simulink model "GPS_Constellation"  (R2018a)
settings: Solver=ode4  StartTime=0  StopTime=time_end  FixedStep=time_step  RelTol=1e-15  AbsTol=1e-15
values from neighbouring files (symbols this model uses):
  c = 299792458    [FFNAV_GPS_Params.mat]    (also in FFNAV_RunGPS.m; Test_GPS_Relativistic.m; Test_Klobuchar_Paper.m)
  GPS_COE = [4.6796815102 2.82369838363 0.203784643463 0.729652347089 1.65659671282 1.15813067845 3.02528391224 5.41010180216 3.56703411206 1.95260455396 0.205879038565 5.92829005708 ... (162 elements, 27x6)]    [FFNAV_GPS_Params.mat]    (also in FFNAV_RunGPS.m = [  268.126*deg2rad    SMA_GPS   ECC_GPS   INC_GPS   357.734*)
  mu = 398600441800000    [FFNAV_GPS_Params.mat]    (also in FFNAV_RunGPS.m; Test_GPS_Relativistic.m = 398600500000000)
undefined symbols (not defined in the file or in its folder): COE_chaser, COE_target
libraries: dspmtrx3 x27
(part 2 of 3)

== matlab function GPS_Constellation/GPS A1 /Orbital Mechanics/Orbital Mechanics ==
  data: v_ECI output; COE input; r_ECI output; mu parameter
 function [v_ECI,r_ECI] = Orb_Mech(COE, mu)
% ========================================================================
% Description: This funciton calculates the initial r and v vectors, 
% given the provided classiclal orbital elements defined in the
% initialization of the simulation.

%%========================================================================
%Extract COE values
theta       = COE(1);
a           = COE(2);
e           = COE(3);
i           = COE(4);
RAAN        = COE(5);
w           = COE(6);

%%========================================================================
r   = a*(1-e^2)/(1+e*cos(theta));                               %Defining the radius (Eq. 2.32)
p   = a*(1-e^2);                                                %Defining the semilatus rectum (Eq. 2.31)
r_P = [r*cos(theta) r*sin(theta) 0]';                           %(r in perifocal frame - Eq. 2.86) 
v_P = [-sqrt(mu/p)*sin(theta) sqrt(mu/p)*(e+cos(theta)) 0]';    %(v in perifocal frame - Eq. 2.87)

%Rotation Matrix from P to ECI Frame
C_IP = [    cos(RAAN)*cos(w)-sin(RAAN)*cos(i)*sin(w) -cos(RAAN)*sin(w)-sin(RAAN)*cos(i)*cos(w) sin(RAAN)*sin(i);
            sin(RAAN)*cos(w)+cos(RAAN)*cos(i)*sin(w) -sin(RAAN)*sin(w)+cos(RAAN)*cos(i)*cos(w) -cos(RAAN)*sin(i);
                        sin(i)*sin(w)                            sin(i)*cos(w)                       cos(i)  ];

%Definition of ECI Frame
x_ECI   = [1 0 0];
y_ECI   = [0 1 0];
z_ECI   = [0 0 1];
F_ECI   = [x_ECI; y_ECI; z_ECI]; %Reference Frame ECI

%r and v vectors in ECI Frame
r_ECI   = F_ECI*C_IP*r_P;
v_ECI   = F_ECI*C_IP*v_P;

%z_vec_ECI  = cross(r_ECI, v_ECI)/norm(cross(r_ECI, v_ECI));    %Check orientation of z vector
%X_ECI      = [r_ECI v_ECI]';                                   %State Vector in ECI components (Eq. 2.82)

r_mag = norm(r_ECI);
r_hat = r_ECI/r_mag;

end
% ========================================================================

== matlab function GPS_Constellation/GPS B1F/Orbital Mechanics/MATLAB Function1 ==
  data: r input; r_ddot output; mu input
function r_ddot = r_ddot(r, mu)
% ========================================================================
% Description: This function calculates -mu/r^3 *r to propagate the radius
% vector of the orbital motion

r_ddot = -(mu/(norm(r))^3)*r;

end
% ========================================================================

== matlab function GPS_Constellation/GPS B1F/Orbital Mechanics/Orbital Mechanics ==
  data: v_ECI output; COE input; r_ECI output; mu input
 function [v_ECI,r_ECI] = Orb_Mech(COE, mu)
% ========================================================================
% Description: This funciton calculates the initial r and v vectors, 
% given the provided classiclal orbital elements defined in the
% initialization of the simulation.

%%========================================================================
%Extract COE values
theta       = COE(1);
a           = COE(2);
e           = COE(3);
i           = COE(4);
RAAN        = COE(5);
w           = COE(6);

%%========================================================================
r   = a*(1-e^2)/(1+e*cos(theta));                               %Defining the radius (Eq. 2.32)
p   = a*(1-e^2);                                                %Defining the semilatus rectum (Eq. 2.31)
r_P = [r*cos(theta) r*sin(theta) 0]';                           %(r in perifocal frame - Eq. 2.86) 
v_P = [-sqrt(mu/p)*sin(theta) sqrt(mu/p)*(e+cos(theta)) 0]';    %(v in perifocal frame - Eq. 2.87)

%Rotation Matrix from P to ECI Frame
C_IP = [    cos(RAAN)*cos(w)-sin(RAAN)*cos(i)*sin(w) -cos(RAAN)*sin(w)-sin(RAAN)*cos(i)*cos(w) sin(RAAN)*sin(i);
            sin(RAAN)*cos(w)+cos(RAAN)*cos(i)*sin(w) -sin(RAAN)*sin(w)+cos(RAAN)*cos(i)*cos(w) -cos(RAAN)*sin(i);
                        sin(i)*sin(w)                            sin(i)*cos(w)                       cos(i)  ];

%Definition of ECI Frame
x_ECI   = [1 0 0];
y_ECI   = [0 1 0];
z_ECI   = [0 0 1];
F_ECI   = [x_ECI; y_ECI; z_ECI]; %Reference Frame ECI

%r and v vectors in ECI Frame
r_ECI   = F_ECI*C_IP*r_P;
v_ECI   = F_ECI*C_IP*v_P;

%z_vec_ECI  = cross(r_ECI, v_ECI)/norm(cross(r_ECI, v_ECI));    %Check orientation of z vector
%X_ECI      = [r_ECI v_ECI]';                                   %State Vector in ECI components (Eq. 2.82)

r_mag = norm(r_ECI);
r_hat = r_ECI/r_mag;

end
% ========================================================================

== matlab function GPS_Constellation/Orbital Mechanics for Target Spacecraft1/MATLAB Function1 ==
  data: r input; r_ddot output; mu parameter
function r_ddot = r_ddot(r, mu)
% ========================================================================
% Description: This function calculates -mu/r^3 *r to propagate the radius
% vector of the orbital motion

r_ddot = -(mu/(norm(r))^3)*r;

end
% ========================================================================

== matlab function GPS_Constellation/Orbital Mechanics for Target Spacecraft1/Target Orbital Mechanics ==
  data: v_ECI output; r_ECI output; mu parameter; COE_target parameter
 function [v_ECI,r_ECI] = Orb_Mech(mu, COE_target)
% ========================================================================
% Description: This funciton calculates the initial r and v vectors, 
% given the provided classiclal orbital elements defined in the
% initialization of the simulation.

%%========================================================================
%Extract COE values
theta       = COE_target(1);
a           = COE_target(2);
e           = COE_target(3);
i           = COE_target(4);
RAAN        = COE_target(5);
w           = COE_target(6);

%%========================================================================
r   = a*(1-e^2)/(1+e*cos(theta));                               %Defining the radius (Eq. 2.32)
p   = a*(1-e^2);                                                %Defining the semilatus rectum (Eq. 2.31)
r_P = [r*cos(theta) r*sin(theta) 0]';                           %(r in perifocal frame - Eq. 2.86) 
v_P = [-sqrt(mu/p)*sin(theta) sqrt(mu/p)*(e+cos(theta)) 0]';    %(v in perifocal frame - Eq. 2.87)

%Rotation Matrix from P to ECI Frame
C_IP = [    cos(RAAN)*cos(w)-sin(RAAN)*cos(i)*sin(w) -cos(RAAN)*sin(w)-sin(RAAN)*cos(i)*cos(w) sin(RAAN)*sin(i);
            sin(RAAN)*cos(w)+cos(RAAN)*cos(i)*sin(w) -sin(RAAN)*sin(w)+cos(RAAN)*cos(i)*cos(w) -cos(RAAN)*sin(i);
                        sin(i)*sin(w)                            sin(i)*cos(w)                       cos(i)  ];

%Definition of ECI Frame
x_ECI   = [1 0 0];
y_ECI   = [0 1 0];
z_ECI   = [0 0 1];
F_ECI   = [x_ECI; y_ECI; z_ECI]; %Reference Frame ECI

%r and v vectors in ECI Frame
r_ECI   = F_ECI*C_IP*r_P;
v_ECI   = F_ECI*C_IP*v_P;

%z_vec_ECI  = cross(r_ECI, v_ECI)/norm(cross(r_ECI, v_ECI));    %Check orientation of z vector
%X_ECI      = [r_ECI v_ECI]';                                   %State Vector in ECI components (Eq. 2.82)

r_mag = norm(r_ECI);
r_hat = r_ECI/r_mag;

end
% ========================================================================

== matlab function GPS_Constellation/GPS A3/Orbital Mechanics/MATLAB Function1 ==
  data: r input; r_ddot output; mu input
function r_ddot = r_ddot(r, mu)
% ========================================================================
% Description: This function calculates -mu/r^3 *r to propagate the radius
% vector of the orbital motion

r_ddot = -(mu/(norm(r))^3)*r;

end
% ========================================================================

== matlab function GPS_Constellation/GPS A3/Orbital Mechanics/Orbital Mechanics ==
  data: v_ECI output; COE input; r_ECI output; mu input
 function [v_ECI,r_ECI] = Orb_Mech(COE, mu)
% ========================================================================
% Description: This funciton calculates the initial r and v vectors, 
% given the provided classiclal orbital elements defined in the
% initialization of the simulation.

%%========================================================================
%Extract COE values
theta       = COE(1);
a           = COE(2);
e           = COE(3);
i           = COE(4);
RAAN        = COE(5);
w           = COE(6);

%%========================================================================
r   = a*(1-e^2)/(1+e*cos(theta));                               %Defining the radius (Eq. 2.32)
p   = a*(1-e^2);                                                %Defining the semilatus rectum (Eq. 2.31)
r_P = [r*cos(theta) r*sin(theta) 0]';                           %(r in perifocal frame - Eq. 2.86) 
v_P = [-sqrt(mu/p)*sin(theta) sqrt(mu/p)*(e+cos(theta)) 0]';    %(v in perifocal frame - Eq. 2.87)

%Rotation Matrix from P to ECI Frame
C_IP = [    cos(RAAN)*cos(w)-sin(RAAN)*cos(i)*sin(w) -cos(RAAN)*sin(w)-sin(RAAN)*cos(i)*cos(w) sin(RAAN)*sin(i);
            sin(RAAN)*cos(w)+cos(RAAN)*cos(i)*sin(w) -sin(RAAN)*sin(w)+cos(RAAN)*cos(i)*cos(w) -cos(RAAN)*sin(i);
                        sin(i)*sin(w)                            sin(i)*cos(w)                       cos(i)  ];

%Definition of ECI Frame
x_ECI   = [1 0 0];
y_ECI   = [0 1 0];
z_ECI   = [0 0 1];
F_ECI   = [x_ECI; y_ECI; z_ECI]; %Reference Frame ECI

%r and v vectors in ECI Frame
r_ECI   = F_ECI*C_IP*r_P;
v_ECI   = F_ECI*C_IP*v_P;

%z_vec_ECI  = cross(r_ECI, v_ECI)/norm(cross(r_ECI, v_ECI));    %Check orientation of z vector
%X_ECI      = [r_ECI v_ECI]';                                   %State Vector in ECI components (Eq. 2.82)

r_mag = norm(r_ECI);
r_hat = r_ECI/r_mag;

end
% ========================================================================

== matlab function GPS_Constellation/GPS A4/Orbital Mechanics/MATLAB Function1 ==
  data: r input; r_ddot output; mu input
function r_ddot = r_ddot(r, mu)
% ========================================================================
% Description: This function calculates -mu/r^3 *r to propagate the radius
% vector of the orbital motion

r_ddot = -(mu/(norm(r))^3)*r;

end
% ========================================================================

== matlab function GPS_Constellation/GPS A4/Orbital Mechanics/Orbital Mechanics ==
  data: v_ECI output; COE input; r_ECI output; mu input
 function [v_ECI,r_ECI] = Orb_Mech(COE, mu)
% ========================================================================
% Description: This funciton calculates the initial r and v vectors, 
% given the provided classiclal orbital elements defined in the
% initialization of the simulation.

%%========================================================================
%Extract COE values
theta       = COE(1);
a           = COE(2);
e           = COE(3);
i           = COE(4);
RAAN        = COE(5);
w           = COE(6);

%%========================================================================
r   = a*(1-e^2)/(1+e*cos(theta));                               %Defining the radius (Eq. 2.32)
p   = a*(1-e^2);                                                %Defining the semilatus rectum (Eq. 2.31)
r_P = [r*cos(theta) r*sin(theta) 0]';                           %(r in perifocal frame - Eq. 2.86) 
v_P = [-sqrt(mu/p)*sin(theta) sqrt(mu/p)*(e+cos(theta)) 0]';    %(v in perifocal frame - Eq. 2.87)

%Rotation Matrix from P to ECI Frame
C_IP = [    cos(RAAN)*cos(w)-sin(RAAN)*cos(i)*sin(w) -cos(RAAN)*sin(w)-sin(RAAN)*cos(i)*cos(w) sin(RAAN)*sin(i);
            sin(RAAN)*cos(w)+cos(RAAN)*cos(i)*sin(w) -sin(RAAN)*sin(w)+cos(RAAN)*cos(i)*cos(w) -cos(RAAN)*sin(i);
                        sin(i)*sin(w)                            sin(i)*cos(w)                       cos(i)  ];

%Definition of ECI Frame
x_ECI   = [1 0 0];
y_ECI   = [0 1 0];
z_ECI   = [0 0 1];
F_ECI   = [x_ECI; y_ECI; z_ECI]; %Reference Frame ECI

%r and v vectors in ECI Frame
r_ECI   = F_ECI*C_IP*r_P;
v_ECI   = F_ECI*C_IP*v_P;

%z_vec_ECI  = cross(r_ECI, v_ECI)/norm(cross(r_ECI, v_ECI));    %Check orientation of z vector
%X_ECI      = [r_ECI v_ECI]';                                   %State Vector in ECI components (Eq. 2.82)

r_mag = norm(r_ECI);
r_hat = r_ECI/r_mag;

end
% ========================================================================

== matlab function GPS_Constellation/GPS B1A/Orbital Mechanics/MATLAB Function1 ==
  data: r input; r_ddot output; mu input
function r_ddot = r_ddot(r, mu)
% ========================================================================
% Description: This function calculates -mu/r^3 *r to propagate the radius
% vector of the orbital motion

r_ddot = -(mu/(norm(r))^3)*r;

end
% ========================================================================

== matlab function GPS_Constellation/GPS B1A/Orbital Mechanics/Orbital Mechanics ==
  data: v_ECI output; COE input; r_ECI output; mu input
 function [v_ECI,r_ECI] = Orb_Mech(COE, mu)
% ========================================================================
% Description: This funciton calculates the initial r and v vectors, 
% given the provided classiclal orbital elements defined in the
% initialization of the simulation.

%%========================================================================
%Extract COE values
theta       = COE(1);
a           = COE(2);
e           = COE(3);
i           = COE(4);
RAAN        = COE(5);
w           = COE(6);

%%========================================================================
r   = a*(1-e^2)/(1+e*cos(theta));                               %Defining the radius (Eq. 2.32)
p   = a*(1-e^2);                                                %Defining the semilatus rectum (Eq. 2.31)
r_P = [r*cos(theta) r*sin(theta) 0]';                           %(r in perifocal frame - Eq. 2.86) 
v_P = [-sqrt(mu/p)*sin(theta) sqrt(mu/p)*(e+cos(theta)) 0]';    %(v in perifocal frame - Eq. 2.87)

%Rotation Matrix from P to ECI Frame
C_IP = [    cos(RAAN)*cos(w)-sin(RAAN)*cos(i)*sin(w) -cos(RAAN)*sin(w)-sin(RAAN)*cos(i)*cos(w) sin(RAAN)*sin(i);
            sin(RAAN)*cos(w)+cos(RAAN)*cos(i)*sin(w) -sin(RAAN)*sin(w)+cos(RAAN)*cos(i)*cos(w) -cos(RAAN)*sin(i);
                        sin(i)*sin(w)                            sin(i)*cos(w)                       cos(i)  ];

%Definition of ECI Frame
x_ECI   = [1 0 0];
y_ECI   = [0 1 0];
z_ECI   = [0 0 1];
F_ECI   = [x_ECI; y_ECI; z_ECI]; %Reference Frame ECI

%r and v vectors in ECI Frame
r_ECI   = F_ECI*C_IP*r_P;
v_ECI   = F_ECI*C_IP*v_P;

%z_vec_ECI  = cross(r_ECI, v_ECI)/norm(cross(r_ECI, v_ECI));    %Check orientation of z vector
%X_ECI      = [r_ECI v_ECI]';                                   %State Vector in ECI components (Eq. 2.82)

r_mag = norm(r_ECI);
r_hat = r_ECI/r_mag;

end
% ========================================================================

== matlab function GPS_Constellation/GPS B2/Orbital Mechanics/MATLAB Function1 ==
  data: r input; r_ddot output; mu input
function r_ddot = r_ddot(r, mu)
% ========================================================================
% Description: This function calculates -mu/r^3 *r to propagate the radius
% vector of the orbital motion

r_ddot = -(mu/(norm(r))^3)*r;

end
% ========================================================================

== matlab function GPS_Constellation/GPS B2/Orbital Mechanics/Orbital Mechanics ==
  data: v_ECI output; COE input; r_ECI output; mu input
 function [v_ECI,r_ECI] = Orb_Mech(COE, mu)
% ========================================================================
% Description: This funciton calculates the initial r and v vectors, 
% given the provided classiclal orbital elements defined in the
% initialization of the simulation.

%%========================================================================
%Extract COE values
theta       = COE(1);
a           = COE(2);
e           = COE(3);
i           = COE(4);
RAAN        = COE(5);
w           = COE(6);

%%========================================================================
r   = a*(1-e^2)/(1+e*cos(theta));                               %Defining the radius (Eq. 2.32)
p   = a*(1-e^2);                                                %Defining the semilatus rectum (Eq. 2.31)
r_P = [r*cos(theta) r*sin(theta) 0]';                           %(r in perifocal frame - Eq. 2.86) 
v_P = [-sqrt(mu/p)*sin(theta) sqrt(mu/p)*(e+cos(theta)) 0]';    %(v in perifocal frame - Eq. 2.87)

%Rotation Matrix from P to ECI Frame
C_IP = [    cos(RAAN)*cos(w)-sin(RAAN)*cos(i)*sin(w) -cos(RAAN)*sin(w)-sin(RAAN)*cos(i)*cos(w) sin(RAAN)*sin(i);
            sin(RAAN)*cos(w)+cos(RAAN)*cos(i)*sin(w) -sin(RAAN)*sin(w)+cos(RAAN)*cos(i)*cos(w) -cos(RAAN)*sin(i);
                        sin(i)*sin(w)                            sin(i)*cos(w)                       cos(i)  ];

%Definition of ECI Frame
x_ECI   = [1 0 0];
y_ECI   = [0 1 0];
z_ECI   = [0 0 1];
F_ECI   = [x_ECI; y_ECI; z_ECI]; %Reference Frame ECI

%r and v vectors in ECI Frame
r_ECI   = F_ECI*C_IP*r_P;
v_ECI   = F_ECI*C_IP*v_P;

%z_vec_ECI  = cross(r_ECI, v_ECI)/norm(cross(r_ECI, v_ECI));    %Check orientation of z vector
%X_ECI      = [r_ECI v_ECI]';                                   %State Vector in ECI components (Eq. 2.82)

r_mag = norm(r_ECI);
r_hat = r_ECI/r_mag;

end
% ========================================================================

== matlab function GPS_Constellation/GPS B3/Orbital Mechanics/MATLAB Function1 ==
  data: r input; r_ddot output; mu input
function r_ddot = r_ddot(r, mu)
% ========================================================================
% Description: This function calculates -mu/r^3 *r to propagate the radius
% vector of the orbital motion

r_ddot = -(mu/(norm(r))^3)*r;

end
% ========================================================================

== matlab function GPS_Constellation/GPS B3/Orbital Mechanics/Orbital Mechanics ==
  data: v_ECI output; COE input; r_ECI output; mu input
 function [v_ECI,r_ECI] = Orb_Mech(COE, mu)
% ========================================================================
% Description: This funciton calculates the initial r and v vectors, 
% given the provided classiclal orbital elements defined in the
% initialization of the simulation.

%%========================================================================
%Extract COE values
theta       = COE(1);
a           = COE(2);
e           = COE(3);
i           = COE(4);
RAAN        = COE(5);
w           = COE(6);

%%========================================================================
r   = a*(1-e^2)/(1+e*cos(theta));                               %Defining the radius (Eq. 2.32)
p   = a*(1-e^2);                                                %Defining the semilatus rectum (Eq. 2.31)
r_P = [r*cos(theta) r*sin(theta) 0]';                           %(r in perifocal frame - Eq. 2.86) 
v_P = [-sqrt(mu/p)*sin(theta) sqrt(mu/p)*(e+cos(theta)) 0]';    %(v in perifocal frame - Eq. 2.87)

%Rotation Matrix from P to ECI Frame
C_IP = [    cos(RAAN)*cos(w)-sin(RAAN)*cos(i)*sin(w) -cos(RAAN)*sin(w)-sin(RAAN)*cos(i)*cos(w) sin(RAAN)*sin(i);
            sin(RAAN)*cos(w)+cos(RAAN)*cos(i)*sin(w) -sin(RAAN)*sin(w)+cos(RAAN)*cos(i)*cos(w) -cos(RAAN)*sin(i);
                        sin(i)*sin(w)                            sin(i)*cos(w)                       cos(i)  ];

%Definition of ECI Frame
x_ECI   = [1 0 0];
y_ECI   = [0 1 0];
z_ECI   = [0 0 1];
F_ECI   = [x_ECI; y_ECI; z_ECI]; %Reference Frame ECI

%r and v vectors in ECI Frame
r_ECI   = F_ECI*C_IP*r_P;
v_ECI   = F_ECI*C_IP*v_P;

%z_vec_ECI  = cross(r_ECI, v_ECI)/norm(cross(r_ECI, v_ECI));    %Check orientation of z vector
%X_ECI      = [r_ECI v_ECI]';                                   %State Vector in ECI components (Eq. 2.82)

r_mag = norm(r_ECI);
r_hat = r_ECI/r_mag;

end
% ========================================================================

== matlab function GPS_Constellation/GPS B4/Orbital Mechanics/MATLAB Function1 ==
  data: r input; r_ddot output; mu input
function r_ddot = r_ddot(r, mu)
% ========================================================================
% Description: This function calculates -mu/r^3 *r to propagate the radius
% vector of the orbital motion

r_ddot = -(mu/(norm(r))^3)*r;

end
% ========================================================================

== matlab function GPS_Constellation/GPS B4/Orbital Mechanics/Orbital Mechanics ==
  data: v_ECI output; COE input; r_ECI output; mu input
 function [v_ECI,r_ECI] = Orb_Mech(COE, mu)
% ========================================================================
% Description: This funciton calculates the initial r and v vectors, 
% given the provided classiclal orbital elements defined in the
% initialization of the simulation.

%%========================================================================
%Extract COE values
theta       = COE(1);
a           = COE(2);
e           = COE(3);
i           = COE(4);
RAAN        = COE(5);
w           = COE(6);

%%========================================================================
r   = a*(1-e^2)/(1+e*cos(theta));                               %Defining the radius (Eq. 2.32)
p   = a*(1-e^2);                                                %Defining the semilatus rectum (Eq. 2.31)
r_P = [r*cos(theta) r*sin(theta) 0]';                           %(r in perifocal frame - Eq. 2.86) 
v_P = [-sqrt(mu/p)*sin(theta) sqrt(mu/p)*(e+cos(theta)) 0]';    %(v in perifocal frame - Eq. 2.87)

%Rotation Matrix from P to ECI Frame
C_IP = [    cos(RAAN)*cos(w)-sin(RAAN)*cos(i)*sin(w) -cos(RAAN)*sin(w)-sin(RAAN)*cos(i)*cos(w) sin(RAAN)*sin(i);
            sin(RAAN)*cos(w)+cos(RAAN)*cos(i)*sin(w) -sin(RAAN)*sin(w)+cos(RAAN)*cos(i)*cos(w) -cos(RAAN)*sin(i);
                        sin(i)*sin(w)                            sin(i)*cos(w)                       cos(i)  ];

%Definition of ECI Frame
x_ECI   = [1 0 0];
y_ECI   = [0 1 0];
z_ECI   = [0 0 1];
F_ECI   = [x_ECI; y_ECI; z_ECI]; %Reference Frame ECI

%r and v vectors in ECI Frame
r_ECI   = F_ECI*C_IP*r_P;
v_ECI   = F_ECI*C_IP*v_P;

%z_vec_ECI  = cross(r_ECI, v_ECI)/norm(cross(r_ECI, v_ECI));    %Check orientation of z vector
%X_ECI      = [r_ECI v_ECI]';                                   %State Vector in ECI components (Eq. 2.82)

r_mag = norm(r_ECI);
r_hat = r_ECI/r_mag;

end
% ========================================================================

== matlab function GPS_Constellation/GPS C3/Orbital Mechanics/MATLAB Function1 ==
  data: r input; r_ddot output; mu input
function r_ddot = r_ddot(r, mu)
% ========================================================================
% Description: This function calculates -mu/r^3 *r to propagate the radius
% vector of the orbital motion

r_ddot = -(mu/(norm(r))^3)*r;

end
% ========================================================================

== matlab function GPS_Constellation/GPS C3/Orbital Mechanics/Orbital Mechanics ==
  data: v_ECI output; COE input; r_ECI output; mu input
 function [v_ECI,r_ECI] = Orb_Mech(COE, mu)
% ========================================================================
% Description: This funciton calculates the initial r and v vectors, 
% given the provided classiclal orbital elements defined in the
% initialization of the simulation.

%%========================================================================
%Extract COE values
theta       = COE(1);
a           = COE(2);
e           = COE(3);
i           = COE(4);
RAAN        = COE(5);
w           = COE(6);

%%========================================================================
r   = a*(1-e^2)/(1+e*cos(theta));                               %Defining the radius (Eq. 2.32)
p   = a*(1-e^2);                                                %Defining the semilatus rectum (Eq. 2.31)
r_P = [r*cos(theta) r*sin(theta) 0]';                           %(r in perifocal frame - Eq. 2.86) 
v_P = [-sqrt(mu/p)*sin(theta) sqrt(mu/p)*(e+cos(theta)) 0]';    %(v in perifocal frame - Eq. 2.87)

%Rotation Matrix from P to ECI Frame
C_IP = [    cos(RAAN)*cos(w)-sin(RAAN)*cos(i)*sin(w) -cos(RAAN)*sin(w)-sin(RAAN)*cos(i)*cos(w) sin(RAAN)*sin(i);
            sin(RAAN)*cos(w)+cos(RAAN)*cos(i)*sin(w) -sin(RAAN)*sin(w)+cos(RAAN)*cos(i)*cos(w) -cos(RAAN)*sin(i);
                        sin(i)*sin(w)                            sin(i)*cos(w)                       cos(i)  ];

%Definition of ECI Frame
x_ECI   = [1 0 0];
y_ECI   = [0 1 0];
z_ECI   = [0 0 1];
F_ECI   = [x_ECI; y_ECI; z_ECI]; %Reference Frame ECI

%r and v vectors in ECI Frame
r_ECI   = F_ECI*C_IP*r_P;
v_ECI   = F_ECI*C_IP*v_P;

%z_vec_ECI  = cross(r_ECI, v_ECI)/norm(cross(r_ECI, v_ECI));    %Check orientation of z vector
%X_ECI      = [r_ECI v_ECI]';                                   %State Vector in ECI components (Eq. 2.82)

r_mag = norm(r_ECI);
r_hat = r_ECI/r_mag;

end
% ========================================================================

== matlab function GPS_Constellation/GPS C2/Orbital Mechanics/MATLAB Function1 ==
  data: r input; r_ddot output; mu input
function r_ddot = r_ddot(r, mu)
% ========================================================================
% Description: This function calculates -mu/r^3 *r to propagate the radius
% vector of the orbital motion

r_ddot = -(mu/(norm(r))^3)*r;

end
% ========================================================================

== matlab function GPS_Constellation/GPS C2/Orbital Mechanics/Orbital Mechanics ==
  data: v_ECI output; COE input; r_ECI output; mu input
 function [v_ECI,r_ECI] = Orb_Mech(COE, mu)
% ========================================================================
% Description: This funciton calculates the initial r and v vectors, 
% given the provided classiclal orbital elements defined in the
% initialization of the simulation.

%%========================================================================
%Extract COE values
theta       = COE(1);
a           = COE(2);
e           = COE(3);
i           = COE(4);
RAAN        = COE(5);
w           = COE(6);

%%========================================================================
r   = a*(1-e^2)/(1+e*cos(theta));                               %Defining the radius (Eq. 2.32)
p   = a*(1-e^2);                                                %Defining the semilatus rectum (Eq. 2.31)
r_P = [r*cos(theta) r*sin(theta) 0]';                           %(r in perifocal frame - Eq. 2.86) 
v_P = [-sqrt(mu/p)*sin(theta) sqrt(mu/p)*(e+cos(theta)) 0]';    %(v in perifocal frame - Eq. 2.87)

%Rotation Matrix from P to ECI Frame
C_IP = [    cos(RAAN)*cos(w)-sin(RAAN)*cos(i)*sin(w) -cos(RAAN)*sin(w)-sin(RAAN)*cos(i)*cos(w) sin(RAAN)*sin(i);
            sin(RAAN)*cos(w)+cos(RAAN)*cos(i)*sin(w) -sin(RAAN)*sin(w)+cos(RAAN)*cos(i)*cos(w) -cos(RAAN)*sin(i);
                        sin(i)*sin(w)                            sin(i)*cos(w)                       cos(i)  ];

%Definition of ECI Frame
x_ECI   = [1 0 0];
y_ECI   = [0 1 0];
z_ECI   = [0 0 1];
F_ECI   = [x_ECI; y_ECI; z_ECI]; %Reference Frame ECI

%r and v vectors in ECI Frame
r_ECI   = F_ECI*C_IP*r_P;
v_ECI   = F_ECI*C_IP*v_P;

%z_vec_ECI  = cross(r_ECI, v_ECI)/norm(cross(r_ECI, v_ECI));    %Check orientation of z vector
%X_ECI      = [r_ECI v_ECI]';                                   %State Vector in ECI components (Eq. 2.82)

r_mag = norm(r_ECI);
r_hat = r_ECI/r_mag;

end
% ========================================================================

== matlab function GPS_Constellation/GPS C1/Orbital Mechanics/MATLAB Function1 ==
  data: r input; r_ddot output; mu input
function r_ddot = r_ddot(r, mu)
% ========================================================================
% Description: This function calculates -mu/r^3 *r to propagate the radius
% vector of the orbital motion

r_ddot = -(mu/(norm(r))^3)*r;

end
% ========================================================================

== matlab function GPS_Constellation/GPS C1/Orbital Mechanics/Orbital Mechanics ==
  data: v_ECI output; COE input; r_ECI output; mu input
 function [v_ECI,r_ECI] = Orb_Mech(COE, mu)
% ========================================================================
% Description: This funciton calculates the initial r and v vectors, 
% given the provided classiclal orbital elements defined in the
% initialization of the simulation.

%%========================================================================
%Extract COE values
theta       = COE(1);
a           = COE(2);
e           = COE(3);
i           = COE(4);
RAAN        = COE(5);
w           = COE(6);

%%========================================================================
r   = a*(1-e^2)/(1+e*cos(theta));                               %Defining the radius (Eq. 2.32)
p   = a*(1-e^2);                                                %Defining the semilatus rectum (Eq. 2.31)
r_P = [r*cos(theta) r*sin(theta) 0]';                           %(r in perifocal frame - Eq. 2.86) 
v_P = [-sqrt(mu/p)*sin(theta) sqrt(mu/p)*(e+cos(theta)) 0]';    %(v in perifocal frame - Eq. 2.87)

%Rotation Matrix from P to ECI Frame
C_IP = [    cos(RAAN)*cos(w)-sin(RAAN)*cos(i)*sin(w) -cos(RAAN)*sin(w)-sin(RAAN)*cos(i)*cos(w) sin(RAAN)*sin(i);
            sin(RAAN)*cos(w)+cos(RAAN)*cos(i)*sin(w) -sin(RAAN)*sin(w)+cos(RAAN)*cos(i)*cos(w) -cos(RAAN)*sin(i);
                        sin(i)*sin(w)                            sin(i)*cos(w)                       cos(i)  ];

%Definition of ECI Frame
x_ECI   = [1 0 0];
y_ECI   = [0 1 0];
z_ECI   = [0 0 1];
F_ECI   = [x_ECI; y_ECI; z_ECI]; %Reference Frame ECI

%r and v vectors in ECI Frame
r_ECI   = F_ECI*C_IP*r_P;
v_ECI   = F_ECI*C_IP*v_P;

%z_vec_ECI  = cross(r_ECI, v_ECI)/norm(cross(r_ECI, v_ECI));    %Check orientation of z vector
%X_ECI      = [r_ECI v_ECI]';                                   %State Vector in ECI components (Eq. 2.82)

r_mag = norm(r_ECI);
r_hat = r_ECI/r_mag;

end
% ========================================================================

== matlab function GPS_Constellation/GPS C4/Orbital Mechanics/MATLAB Function1 ==
  data: r input; r_ddot output; mu input
function r_ddot = r_ddot(r, mu)
% ========================================================================
% Description: This function calculates -mu/r^3 *r to propagate the radius
% vector of the orbital motion

r_ddot = -(mu/(norm(r))^3)*r;

end
% ========================================================================

== matlab function GPS_Constellation/GPS C4/Orbital Mechanics/Orbital Mechanics ==
  data: v_ECI output; COE input; r_ECI output; mu input
 function [v_ECI,r_ECI] = Orb_Mech(COE, mu)
% ========================================================================
% Description: This funciton calculates the initial r and v vectors, 
% given the provided classiclal orbital elements defined in the
% initialization of the simulation.

%%========================================================================
%Extract COE values
theta       = COE(1);
a           = COE(2);
e           = COE(3);
i           = COE(4);
RAAN        = COE(5);
w           = COE(6);

%%========================================================================
r   = a*(1-e^2)/(1+e*cos(theta));                               %Defining the radius (Eq. 2.32)
p   = a*(1-e^2);                                                %Defining the semilatus rectum (Eq. 2.31)
r_P = [r*cos(theta) r*sin(theta) 0]';                           %(r in perifocal frame - Eq. 2.86) 
v_P = [-sqrt(mu/p)*sin(theta) sqrt(mu/p)*(e+cos(theta)) 0]';    %(v in perifocal frame - Eq. 2.87)

%Rotation Matrix from P to ECI Frame
C_IP = [    cos(RAAN)*cos(w)-sin(RAAN)*cos(i)*sin(w) -cos(RAAN)*sin(w)-sin(RAAN)*cos(i)*cos(w) sin(RAAN)*sin(i);
            sin(RAAN)*cos(w)+cos(RAAN)*cos(i)*sin(w) -sin(RAAN)*sin(w)+cos(RAAN)*cos(i)*cos(w) -cos(RAAN)*sin(i);
                        sin(i)*sin(w)                            sin(i)*cos(w)                       cos(i)  ];

%Definition of ECI Frame
x_ECI   = [1 0 0];
y_ECI   = [0 1 0];
z_ECI   = [0 0 1];
F_ECI   = [x_ECI; y_ECI; z_ECI]; %Reference Frame ECI

%r and v vectors in ECI Frame
r_ECI   = F_ECI*C_IP*r_P;
v_ECI   = F_ECI*C_IP*v_P;

%z_vec_ECI  = cross(r_ECI, v_ECI)/norm(cross(r_ECI, v_ECI));    %Check orientation of z vector
%X_ECI      = [r_ECI v_ECI]';                                   %State Vector in ECI components (Eq. 2.82)

r_mag = norm(r_ECI);
r_hat = r_ECI/r_mag;

end
% ========================================================================

== matlab function GPS_Constellation/GPS D2A/Orbital Mechanics/MATLAB Function1 ==
  data: r input; r_ddot output; mu input
function r_ddot = r_ddot(r, mu)
% ========================================================================
% Description: This function calculates -mu/r^3 *r to propagate the radius
% vector of the orbital motion

r_ddot = -(mu/(norm(r))^3)*r;

end
% ========================================================================

== matlab function GPS_Constellation/GPS D2A/Orbital Mechanics/Orbital Mechanics ==
  data: v_ECI output; COE input; r_ECI output; mu input
 function [v_ECI,r_ECI] = Orb_Mech(COE, mu)
% ========================================================================
% Description: This funciton calculates the initial r and v vectors, 
% given the provided classiclal orbital elements defined in the
% initialization of the simulation.

%%========================================================================
%Extract COE values
theta       = COE(1);
a           = COE(2);
e           = COE(3);
i           = COE(4);
RAAN        = COE(5);
w           = COE(6);

%%========================================================================
r   = a*(1-e^2)/(1+e*cos(theta));                               %Defining the radius (Eq. 2.32)
p   = a*(1-e^2);                                                %Defining the semilatus rectum (Eq. 2.31)
r_P = [r*cos(theta) r*sin(theta) 0]';                           %(r in perifocal frame - Eq. 2.86) 
v_P = [-sqrt(mu/p)*sin(theta) sqrt(mu/p)*(e+cos(theta)) 0]';    %(v in perifocal frame - Eq. 2.87)

%Rotation Matrix from P to ECI Frame
C_IP = [    cos(RAAN)*cos(w)-sin(RAAN)*cos(i)*sin(w) -cos(RAAN)*sin(w)-sin(RAAN)*cos(i)*cos(w) sin(RAAN)*sin(i);
            sin(RAAN)*cos(w)+cos(RAAN)*cos(i)*sin(w) -sin(RAAN)*sin(w)+cos(RAAN)*cos(i)*cos(w) -cos(RAAN)*sin(i);
                        sin(i)*sin(w)                            sin(i)*cos(w)                       cos(i)  ];

%Definition of ECI Frame
x_ECI   = [1 0 0];
y_ECI   = [0 1 0];
z_ECI   = [0 0 1];
F_ECI   = [x_ECI; y_ECI; z_ECI]; %Reference Frame ECI

%r and v vectors in ECI Frame
r_ECI   = F_ECI*C_IP*r_P;
v_ECI   = F_ECI*C_IP*v_P;

%z_vec_ECI  = cross(r_ECI, v_ECI)/norm(cross(r_ECI, v_ECI));    %Check orientation of z vector
%X_ECI      = [r_ECI v_ECI]';                                   %State Vector in ECI components (Eq. 2.82)

r_mag = norm(r_ECI);
r_hat = r_ECI/r_mag;

end
% ========================================================================

== matlab function GPS_Constellation/GPS D2F/Orbital Mechanics/MATLAB Function1 ==
  data: r input; r_ddot output; mu input
function r_ddot = r_ddot(r, mu)
% ========================================================================
% Description: This function calculates -mu/r^3 *r to propagate the radius
% vector of the orbital motion

r_ddot = -(mu/(norm(r))^3)*r;

end
% ========================================================================

== matlab function GPS_Constellation/GPS D2F/Orbital Mechanics/Orbital Mechanics ==
  data: v_ECI output; COE input; r_ECI output; mu input
 function [v_ECI,r_ECI] = Orb_Mech(COE, mu)
% ========================================================================
% Description: This funciton calculates the initial r and v vectors, 
% given the provided classiclal orbital elements defined in the
% initialization of the simulation.

%%========================================================================
%Extract COE values
theta       = COE(1);
a           = COE(2);
e           = COE(3);
i           = COE(4);
RAAN        = COE(5);
w           = COE(6);

%%========================================================================
r   = a*(1-e^2)/(1+e*cos(theta));                               %Defining the radius (Eq. 2.32)
p   = a*(1-e^2);                                                %Defining the semilatus rectum (Eq. 2.31)
r_P = [r*cos(theta) r*sin(theta) 0]';                           %(r in perifocal frame - Eq. 2.86) 
v_P = [-sqrt(mu/p)*sin(theta) sqrt(mu/p)*(e+cos(theta)) 0]';    %(v in perifocal frame - Eq. 2.87)

%Rotation Matrix from P to ECI Frame
C_IP = [    cos(RAAN)*cos(w)-sin(RAAN)*cos(i)*sin(w) -cos(RAAN)*sin(w)-sin(RAAN)*cos(i)*cos(w) sin(RAAN)*sin(i);
            sin(RAAN)*cos(w)+cos(RAAN)*cos(i)*sin(w) -sin(RAAN)*sin(w)+cos(RAAN)*cos(i)*cos(w) -cos(RAAN)*sin(i);
                        sin(i)*sin(w)                            sin(i)*cos(w)                       cos(i)  ];

%Definition of ECI Frame
x_ECI   = [1 0 0];
y_ECI   = [0 1 0];
z_ECI   = [0 0 1];
F_ECI   = [x_ECI; y_ECI; z_ECI]; %Reference Frame ECI

%r and v vectors in ECI Frame
r_ECI   = F_ECI*C_IP*r_P;
v_ECI   = F_ECI*C_IP*v_P;

%z_vec_ECI  = cross(r_ECI, v_ECI)/norm(cross(r_ECI, v_ECI));    %Check orientation of z vector
%X_ECI      = [r_ECI v_ECI]';                                   %State Vector in ECI components (Eq. 2.82)

r_mag = norm(r_ECI);
r_hat = r_ECI/r_mag;

end
% ========================================================================

== matlab function GPS_Constellation/GPS D1/Orbital Mechanics/MATLAB Function1 ==
  data: r input; r_ddot output; mu input
function r_ddot = r_ddot(r, mu)
% ========================================================================
% Description: This function calculates -mu/r^3 *r to propagate the radius
% vector of the orbital motion

r_ddot = -(mu/(norm(r))^3)*r;

end
% ========================================================================

== matlab function GPS_Constellation/GPS D1/Orbital Mechanics/Orbital Mechanics ==
  data: v_ECI output; COE input; r_ECI output; mu input
 function [v_ECI,r_ECI] = Orb_Mech(COE, mu)
% ========================================================================
% Description: This funciton calculates the initial r and v vectors, 
% given the provided classiclal orbital elements defined in the
% initialization of the simulation.

%%========================================================================
%Extract COE values
theta       = COE(1);
a           = COE(2);
e           = COE(3);
i           = COE(4);
RAAN        = COE(5);
w           = COE(6);

%%========================================================================
r   = a*(1-e^2)/(1+e*cos(theta));                               %Defining the radius (Eq. 2.32)
p   = a*(1-e^2);                                                %Defining the semilatus rectum (Eq. 2.31)
r_P = [r*cos(theta) r*sin(theta) 0]';                           %(r in perifocal frame - Eq. 2.86) 
v_P = [-sqrt(mu/p)*sin(theta) sqrt(mu/p)*(e+cos(theta)) 0]';    %(v in perifocal frame - Eq. 2.87)

%Rotation Matrix from P to ECI Frame
C_IP = [    cos(RAAN)*cos(w)-sin(RAAN)*cos(i)*sin(w) -cos(RAAN)*sin(w)-sin(RAAN)*cos(i)*cos(w) sin(RAAN)*sin(i);
            sin(RAAN)*cos(w)+cos(RAAN)*cos(i)*sin(w) -sin(RAAN)*sin(w)+cos(RAAN)*cos(i)*cos(w) -cos(RAAN)*sin(i);
                        sin(i)*sin(w)                            sin(i)*cos(w)                       cos(i)  ];

%Definition of ECI Frame
x_ECI   = [1 0 0];
y_ECI   = [0 1 0];
z_ECI   = [0 0 1];
F_ECI   = [x_ECI; y_ECI; z_ECI]; %Reference Frame ECI

%r and v vectors in ECI Frame
r_ECI   = F_ECI*C_IP*r_P;
v_ECI   = F_ECI*C_IP*v_P;

%z_vec_ECI  = cross(r_ECI, v_ECI)/norm(cross(r_ECI, v_ECI));    %Check orientation of z vector
%X_ECI      = [r_ECI v_ECI]';                                   %State Vector in ECI components (Eq. 2.82)

r_mag = norm(r_ECI);
r_hat = r_ECI/r_mag;

end
% ========================================================================

== matlab function GPS_Constellation/GPS D3/Orbital Mechanics/MATLAB Function1 ==
  data: r input; r_ddot output; mu input
function r_ddot = r_ddot(r, mu)
% ========================================================================
% Description: This function calculates -mu/r^3 *r to propagate the radius
% vector of the orbital motion

r_ddot = -(mu/(norm(r))^3)*r;

end
% ========================================================================

== matlab function GPS_Constellation/GPS D3/Orbital Mechanics/Orbital Mechanics ==
  data: v_ECI output; COE input; r_ECI output; mu input
 function [v_ECI,r_ECI] = Orb_Mech(COE, mu)
% ========================================================================
% Description: This funciton calculates the initial r and v vectors, 
% given the provided classiclal orbital elements defined in the
% initialization of the simulation.

%%========================================================================
%Extract COE values
theta       = COE(1);
a           = COE(2);
e           = COE(3);
i           = COE(4);
RAAN        = COE(5);
w           = COE(6);

%%========================================================================
r   = a*(1-e^2)/(1+e*cos(theta));                               %Defining the radius (Eq. 2.32)
p   = a*(1-e^2);                                                %Defining the semilatus rectum (Eq. 2.31)
r_P = [r*cos(theta) r*sin(theta) 0]';                           %(r in perifocal frame - Eq. 2.86) 
v_P = [-sqrt(mu/p)*sin(theta) sqrt(mu/p)*(e+cos(theta)) 0]';    %(v in perifocal frame - Eq. 2.87)

%Rotation Matrix from P to ECI Frame
C_IP = [    cos(RAAN)*cos(w)-sin(RAAN)*cos(i)*sin(w) -cos(RAAN)*sin(w)-sin(RAAN)*cos(i)*cos(w) sin(RAAN)*sin(i);
            sin(RAAN)*cos(w)+cos(RAAN)*cos(i)*sin(w) -sin(RAAN)*sin(w)+cos(RAAN)*cos(i)*cos(w) -cos(RAAN)*sin(i);
                        sin(i)*sin(w)                            sin(i)*cos(w)                       cos(i)  ];

%Definition of ECI Frame
x_ECI   = [1 0 0];
y_ECI   = [0 1 0];
z_ECI   = [0 0 1];
F_ECI   = [x_ECI; y_ECI; z_ECI]; %Reference Frame ECI

%r and v vectors in ECI Frame
r_ECI   = F_ECI*C_IP*r_P;
v_ECI   = F_ECI*C_IP*v_P;

%z_vec_ECI  = cross(r_ECI, v_ECI)/norm(cross(r_ECI, v_ECI));    %Check orientation of z vector
%X_ECI      = [r_ECI v_ECI]';                                   %State Vector in ECI components (Eq. 2.82)

r_mag = norm(r_ECI);
r_hat = r_ECI/r_mag;

end
% ========================================================================

== matlab function GPS_Constellation/GPS D4/Orbital Mechanics/MATLAB Function1 ==
  data: r input; r_ddot output; mu input
function r_ddot = r_ddot(r, mu)
% ========================================================================
% Description: This function calculates -mu/r^3 *r to propagate the radius
% vector of the orbital motion

r_ddot = -(mu/(norm(r))^3)*r;

end
% ========================================================================

== matlab function GPS_Constellation/GPS D4/Orbital Mechanics/Orbital Mechanics ==
  data: v_ECI output; COE input; r_ECI output; mu input
 function [v_ECI,r_ECI] = Orb_Mech(COE, mu)
% ========================================================================
% Description: This funciton calculates the initial r and v vectors, 
% given the provided classiclal orbital elements defined in the
% initialization of the simulation.

%%========================================================================
%Extract COE values
theta       = COE(1);
a           = COE(2);
e           = COE(3);
i           = COE(4);
RAAN        = COE(5);
w           = COE(6);

%%========================================================================
r   = a*(1-e^2)/(1+e*cos(theta));                               %Defining the radius (Eq. 2.32)
p   = a*(1-e^2);                                                %Defining the semilatus rectum (Eq. 2.31)
r_P = [r*cos(theta) r*sin(theta) 0]';                           %(r in perifocal frame - Eq. 2.86) 
v_P = [-sqrt(mu/p)*sin(theta) sqrt(mu/p)*(e+cos(theta)) 0]';    %(v in perifocal frame - Eq. 2.87)

%Rotation Matrix from P to ECI Frame
C_IP = [    cos(RAAN)*cos(w)-sin(RAAN)*cos(i)*sin(w) -cos(RAAN)*sin(w)-sin(RAAN)*cos(i)*cos(w) sin(RAAN)*sin(i);
            sin(RAAN)*cos(w)+cos(RAAN)*cos(i)*sin(w) -sin(RAAN)*sin(w)+cos(RAAN)*cos(i)*cos(w) -cos(RAAN)*sin(i);
                        sin(i)*sin(w)                            sin(i)*cos(w)                       cos(i)  ];

%Definition of ECI Frame
x_ECI   = [1 0 0];
y_ECI   = [0 1 0];
z_ECI   = [0 0 1];
F_ECI   = [x_ECI; y_ECI; z_ECI]; %Reference Frame ECI

%r and v vectors in ECI Frame
r_ECI   = F_ECI*C_IP*r_P;
v_ECI   = F_ECI*C_IP*v_P;

%z_vec_ECI  = cross(r_ECI, v_ECI)/norm(cross(r_ECI, v_ECI));    %Check orientation of z vector
%X_ECI      = [r_ECI v_ECI]';                                   %State Vector in ECI components (Eq. 2.82)

r_mag = norm(r_ECI);
r_hat = r_ECI/r_mag;

end
% ========================================================================

== matlab function GPS_Constellation/GPS E1/Orbital Mechanics/MATLAB Function1 ==
  data: r input; r_ddot output; mu input
function r_ddot = r_ddot(r, mu)
% ========================================================================
% Description: This function calculates -mu/r^3 *r to propagate the radius
% vector of the orbital motion

r_ddot = -(mu/(norm(r))^3)*r;

end
% ========================================================================

== matlab function GPS_Constellation/GPS E1/Orbital Mechanics/Orbital Mechanics ==
  data: v_ECI output; COE input; r_ECI output; mu input
 function [v_ECI,r_ECI] = Orb_Mech(COE, mu)
% ========================================================================
% Description: This funciton calculates the initial r and v vectors, 
% given the provided classiclal orbital elements defined in the
% initialization of the simulation.

%%========================================================================
%Extract COE values
theta       = COE(1);
a           = COE(2);
e           = COE(3);
i           = COE(4);
RAAN        = COE(5);
w           = COE(6);

%%========================================================================
r   = a*(1-e^2)/(1+e*cos(theta));                               %Defining the radius (Eq. 2.32)
p   = a*(1-e^2);                                                %Defining the semilatus rectum (Eq. 2.31)
r_P = [r*cos(theta) r*sin(theta) 0]';                           %(r in perifocal frame - Eq. 2.86) 
v_P = [-sqrt(mu/p)*sin(theta) sqrt(mu/p)*(e+cos(theta)) 0]';    %(v in perifocal frame - Eq. 2.87)

%Rotation Matrix from P to ECI Frame
C_IP = [    cos(RAAN)*cos(w)-sin(RAAN)*cos(i)*sin(w) -cos(RAAN)*sin(w)-sin(RAAN)*cos(i)*cos(w) sin(RAAN)*sin(i);
            sin(RAAN)*cos(w)+cos(RAAN)*cos(i)*sin(w) -sin(RAAN)*sin(w)+cos(RAAN)*cos(i)*cos(w) -cos(RAAN)*sin(i);
                        sin(i)*sin(w)                            sin(i)*cos(w)                       cos(i)  ];

%Definition of ECI Frame
x_ECI   = [1 0 0];
y_ECI   = [0 1 0];
z_ECI   = [0 0 1];
F_ECI   = [x_ECI; y_ECI; z_ECI]; %Reference Frame ECI

%r and v vectors in ECI Frame
r_ECI   = F_ECI*C_IP*r_P;
v_ECI   = F_ECI*C_IP*v_P;

%z_vec_ECI  = cross(r_ECI, v_ECI)/norm(cross(r_ECI, v_ECI));    %Check orientation of z vector
%X_ECI      = [r_ECI v_ECI]';                                   %State Vector in ECI components (Eq. 2.82)

r_mag = norm(r_ECI);
r_hat = r_ECI/r_mag;

end
% ========================================================================

== matlab function GPS_Constellation/GPS E2/Orbital Mechanics/MATLAB Function1 ==
  data: r input; r_ddot output; mu input
function r_ddot = r_ddot(r, mu)
% ========================================================================
% Description: This function calculates -mu/r^3 *r to propagate the radius
% vector of the orbital motion

r_ddot = -(mu/(norm(r))^3)*r;

end
% ========================================================================
